simulink model "CONTROLLER_PI"  (R2023b)
settings: Solver=FixedStepAuto  StartTime=0.0  StopTime=inf  FixedStep=0.1  RelTol=1e-3  EnableMultiTasking=on
undefined symbols (not defined in the file or in its folder): Ts
libraries: arduinosensorlib x1, arduinolib x1
settings Model: ExtModeTrigDuration=2  Creator=Cesar Andres  LastModifiedBy=Cesar Andres
settings OptimizationCC: EnhancedBackFolding=on  PassReuseOutputArgsAs=Individual arguments  ZeroExternalMemoryAtStartup=off  ZeroInternalMemoryAtStartup=off  MaxStackSize=64  OptimizeBlockOrder=speed  DifferentSizesBufferReuse=on  OptimizationCustomize=off  EfficientTunableParamExpr=on
settings DebuggingCC: ParameterTunabilityLossMsg=error
settings HardwareCC: ProdBitPerInt=16  ProdBitPerPointer=16  ProdBitPerSizeT=16  ProdBitPerPtrDiffT=16  ProdLargestAtomicFloat=None  ProdWordSize=8  ProdHWDeviceType=Atmel->AVR  UseEmbeddedCoderFeatures=off  UseSimulinkCoderFeatures=off
settings SFSimCC: MATLABDynamicMemAlloc=off
settings RTWCC: Description=Embedded Coder  SystemTargetFile=ert.tlc  HardwareBoard=Arduino Uno  TemplateMakefile=ert_default_tmf  Toolchain=Arduino AVR  BuildConfiguration=Faster Runs
settings CodeAppCC: ForceParamTrailComments=on  IgnoreCustomStorageClasses=off  OperatorAnnotations=on  SimulinkDataObjDesc=on  SFDataObjDesc=on  InsertBlockDesc=on
settings ERTTargetCC: SupportContinuousTime=on  SupportNonInlinedSFcns=on  SupportVariableSizeSignals=on  ExtModeTransport=3  ExtModeStaticAlloc=on  ExtModeAutomaticAllocSize=off  ExtModeStaticAllocSize=250  ExtModeMexFile=ext_xcp  ExtModeIntrfLevel=Level2 - Open

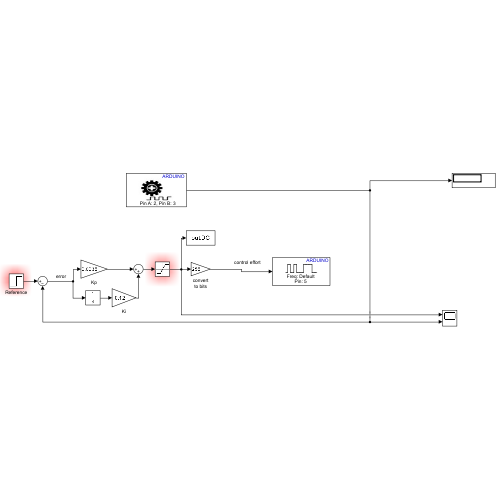
[thumbnail: Simulink's stored preview of the top-level diagram]
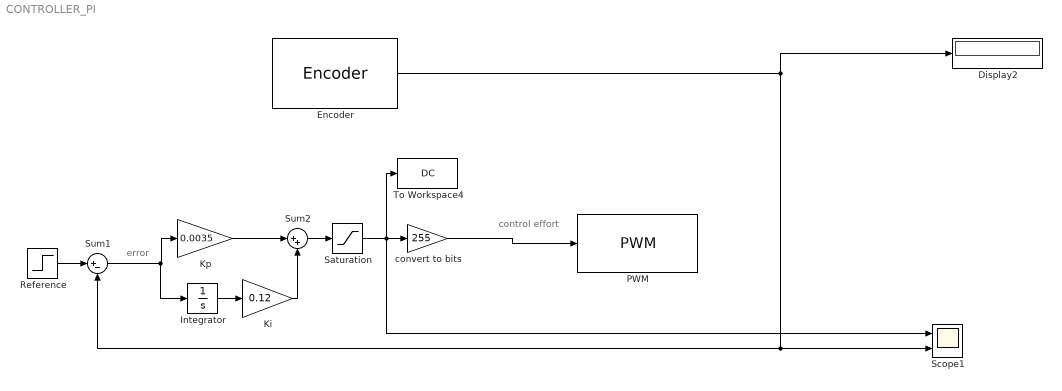
== system CONTROLLER_PI ==
  note: control effort
  note: error
  Display2 : Display
  Encoder : arduinosensorlib/Encoder  InputA=2  InputB=3  Mode=No reset  SampleTime=-1
  Integrator : Integrator
  Ki : Gain  Gain=0.12
  "Kp " : Gain  Gain=0.0035
  PWM : arduinolib/PWM  pinNumber=5  frequencyType=Default  desiredFrequency=490.2  achievableFrequency=490.2
  Reference : Step  After=130  SampleTime=Ts
  Saturation : Saturate  UpperLimit=1  LowerLimit=0  SampleTime=Ts
  Scope1 : Scope  NumInputPorts=2
  Sum1 : Sum  Inputs=|+-
  Sum2 : Sum  Inputs=|++
  To Workspace4 : ToWorkspace  VariableName=DC  SaveFormat=Timeseries  SampleTime=-1
  convert to bits : Gain  Gain=255
  wires:
  Sum1/1 -> Integrator/1, "Kp "/1
  "Kp "/1 -> Sum2/1
  Reference/1 -> Sum1/1
  Encoder/1 -> Display2/1, Sum1/2, Scope1/2
  Ki/1 -> Sum2/2
  Saturation/1 -> Scope1/1, To Workspace4/1, convert to bits/1
  Sum2/1 -> Saturation/1
  convert to bits/1 -> PWM/1
  Integrator/1 -> Ki/1
